simulink model "linea_system"  (R2020a)
settings: Solver=VariableStepAuto  StartTime=0.0  StopTime=1000  RelTol=1e-3
settings Model: Creator=啊包PC  LastModifiedBy=啊包PC

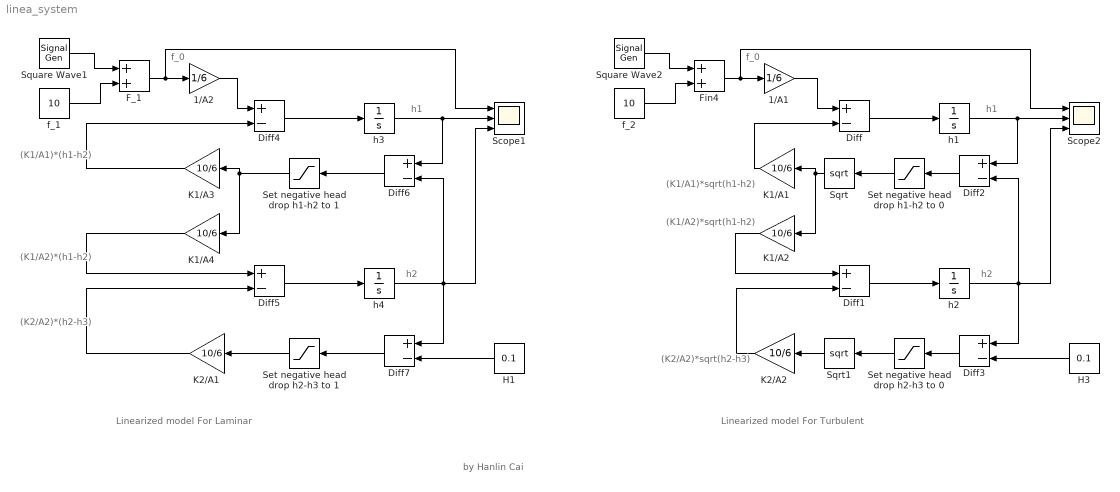
== system linea_system ==
  note: f_0
  note: (K1/A1)*(h1-h2)
  note: h1
  note: (K2/A2)*(h2-h3)
  note: h2
  note: (K1/A2)*(h1-h2)
  note: Linearized model For Turbulent
  note: (K1/A2)*sqrt(h1-h2)
  note: by Hanlin Cai
  note: (K1/A1)*sqrt(h1-h2)
  note: h1
  note: (K2/A2)*sqrt(h2-h3)
  note: h2
  note: f_0
  note: Linearized model For Laminar
  1/A1 : Gain  Gain=1/6
  1/A2 : Gain  Gain=1/6
  Diff{,1..7} (8 alike) : Sum  Inputs=+-
  F_1 : Sum
  Fin4 : Sum
  H1 : Constant  Value=0.1
  H3 : Constant  Value=0.1
  K1/A{1..4} (4 alike) : Gain  Gain=10/6
  K2/A1 : Gain  Gain=10/6
  K2/A2 : Gain  Gain=10/6
  Scope1 : Scope  NumInputPorts=3
  Scope2 : Scope  NumInputPorts=3
  Set negative head drop h1-h2 to 0 : Saturate  UpperLimit=Inf  LowerLimit=0  ZeroCross=off
  Set negative head drop h1-h2 to 1 : Saturate  UpperLimit=Inf  LowerLimit=0  ZeroCross=off
  Set negative head drop h2-h3 to 0 : Saturate  UpperLimit=Inf  LowerLimit=0  ZeroCross=off
  Set negative head drop h2-h3 to 1 : Saturate  UpperLimit=Inf  LowerLimit=0  ZeroCross=off
  Sqrt : Sqrt  SaturateOnIntegerOverflow=on
  Sqrt1 : Sqrt  SaturateOnIntegerOverflow=on
  Square Wave1 : SignalGenerator  WaveForm=square  Amplitude=0.3*10  Frequency=1/60
  Square Wave2 : SignalGenerator  WaveForm=square  Amplitude=0.3*10  Frequency=1/60
  f_1 : Constant  Value=10
  f_2 : Constant  Value=10
  h{1..4} (4 alike) : Integrator
  wires:
  K1/A4/1 -> Diff5/1
  Set negative head drop h2-h3 to 1/1 -> K2/A1/1
  Diff7/1 -> Set negative head drop h2-h3 to 1/1
  Square Wave1/1 -> F_1/1
  K2/A1/1 -> Diff5/2
  h4/1 -> Diff7/1, Diff6/2, Scope1/3
  F_1/1 -> Scope1/1, 1/A2/1
  H1/1 -> Diff7/2
  Diff6/1 -> Set negative head drop h1-h2 to 1/1
  Diff5/1 -> h4/1
  Diff4/1 -> h3/1
  Set negative head drop h1-h2 to 1/1 -> K1/A4/1, K1/A3/1
  K1/A3/1 -> Diff4/2
  1/A2/1 -> Diff4/1
  f_1/1 -> F_1/2
  h3/1 -> Scope1/2, Diff6/1
  Set negative head drop h1-h2 to 0/1 -> Sqrt/1
  K1/A1/1 -> Diff/2
  K2/A2/1 -> Diff1/2
  h1/1 -> Scope2/2, Diff2/1
  Diff1/1 -> h2/1
  Square Wave2/1 -> Fin4/1
  Diff/1 -> h1/1
  Set negative head drop h2-h3 to 0/1 -> Sqrt1/1
  H3/1 -> Diff3/2
  Sqrt1/1 -> K2/A2/1
  h2/1 -> Diff3/1, Diff2/2, Scope2/3
  Diff2/1 -> Set negative head drop h1-h2 to 0/1
  Sqrt/1 -> K1/A2/1, K1/A1/1
  f_2/1 -> Fin4/2
  K1/A2/1 -> Diff1/1
  Diff3/1 -> Set negative head drop h2-h3 to 0/1
  Fin4/1 -> Scope2/1, 1/A1/1
  1/A1/1 -> Diff/1
